simulink model "gm_gm_hdlcoder_commviterbi"  (R2023b)
settings: Solver=FixedStepDiscrete  StartTime=0.0  StopTime=5000  RelTol=1e-3
InitFcn:
  | EbNo=3;
libraries: commcnvcod2 x2, commrandsrc3 x1, commsink2 x1
Description:
  | Viterbi Decoder Using Simulink(R) Blocks
  | This model shows how to use HDL Coder(TM) to check, generate,
  | and verify HDL for a fixed-point Viterbi decoder model built using Simulink(R) blocks.
settings Model: Creator=The MathWorks, Inc.  LastModifiedBy=bryan
settings SolverCC: AlgebraicLoopSolver=TrustRegion  MaxZcPerStep=1
settings DataIOCC: LimitDataPoints=on  SaveFormat=Array  SaveOutput=off  SignalLogging=off  SaveTime=off  ReturnWorkspaceOutputs=off
settings OptimizationCC: BlockReduction=off  ConditionallyExecuteInputs=off  DefaultParameterBehavior=Inlined  ReuseModelBlockBuffer=off  ExpressionDepthLimit=2147483647  InitFltsAndDblsToZero=on  EfficientMapNaN2IntZero=off  LifeSpan=inf
settings DebuggingCC: AlgebraicLoopMsg=error  SignalResolutionControl=TryResolveAllWithWarning  SolverPrmCheckMsg=warning  InheritedTsInSrcMsg=none  MultiTaskDSMMsg=warning  MultiTaskCondExecSysMsg=none  SingleTaskRateTransMsg=error  IntegerOverflowMsg=none  ParameterPrecisionLossMsg=none  UnconnectedInputMsg=warning  UnconnectedOutputMsg=warning  UnconnectedLineMsg=warning  StateNameClashWarn=warning  SymbolicDimsDataTypeCodeGenerationDiagnostic=none  SFUnexpectedBacktrackingDiag=warning  SFNoUnconditionalDefaultTransitionDiag=warning  SFExecutionAtInitializationDiag=none  IntegerSaturationMsg=none  ArithmeticOperatorsInVariantConditions=warning
settings HardwareCC: ProdBitPerPointer=32  ProdBitPerSizeT=32  ProdBitPerPtrDiffT=32  ProdLargestAtomicFloat=None  ProdIntDivRoundTo=Undefined  ProdEndianess=Unspecified  ProdWordSize=32  ProdHWDeviceType=ASIC/FPGA  ProdEqTarget=off
settings ModelReferenceCC: EnableRefExpFcnMdlSchedulingChecks=on  PropagateSignalLabelsOutOfModel=off
settings SFSimCC: SimUseLocalCustomCode=off  CustomCodeUndefinedFunction=UseInterfaceOnly
settings RTWCC: RTWUseLocalCustomCode=off  DLArmComputeVersion=19.05
settings CodeAppCC: StateflowObjectComments=on
settings GRTTargetCC: TargetLangStandard=C89/C90 (ANSI)  CombineOutputUpdateFcns=off  GRTInterface=on
settings ConfigComp: CovMetricSettings=dw  CovSaveCumulativeToWorkspaceVar=on  CovSaveSingleToWorkspaceVar=on  CovExternalEMLEnable=off  CovSFcnEnable=off

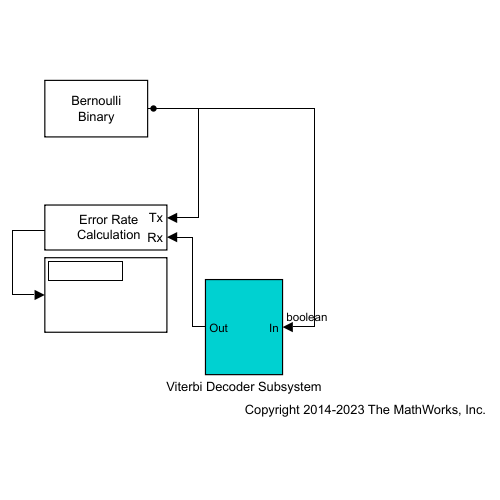
[thumbnail: Simulink's stored preview of the top-level diagram]
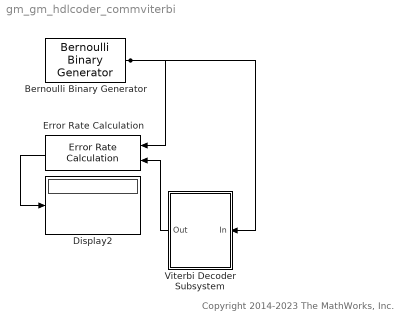
== system gm_gm_hdlcoder_commviterbi ==
  note: Copyright 2014-2023 The MathWorks, Inc.
  Bernoulli Binary Generator : commrandsrc3/Bernoulli Binary Generator  ProbabilityOfZero=0.5  SeedSource=Parameter  Seed=610  SampleTime=1  SamplesPerFrame=1  OutputDataType=boolean  SimulateUsing=Interpreted execution
  Display2 : Display
  Error Rate Calculation : commsink2/Error Rate Calculation  N=32  st_delay=0  cp_mode=Entire frame  subframe=[]  PMode=Port  WsName=BER_Data  RsMode2=off  stop=off  numErr=500  maxBits=1e6
  Viterbi Decoder Subsystem : Subsystem
  wires:
  Bernoulli Binary Generator/1 -> Viterbi Decoder Subsystem/1(In), Error Rate Calculation/1
  Error Rate Calculation/1 -> Display2/1
  Viterbi Decoder Subsystem/1(Out) -> Error Rate Calculation/2

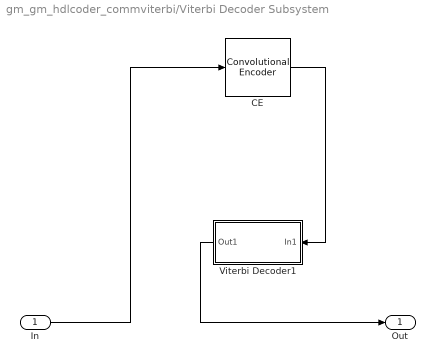
== system gm_gm_hdlcoder_commviterbi/Viterbi Decoder Subsystem ==
  In : Inport  OutDataTypeStr=boolean  PortDimensions=1  SampleTime=1
  CE : commcnvcod2/Convolutional Encoder  trellis=poly2trellis(3,[6 7])  opMode=Continuous  DelayedResetAction=off  hasIniStPort=off  hasFinStPort=off  usePuncVector=off  punctureVector=[1; 1; 0; 1; 0; 1]  reset=Unused parameter value
  Viterbi Decoder1 : Subsystem
  Out : Outport  SampleTime=1  VectorParamsAs1DForOutWhenUnconnected=off
  wires:
  In/1 -> CE/1
  CE/1 -> Viterbi Decoder1/1(In1)
  Viterbi Decoder1/1(Out1) -> Out/1

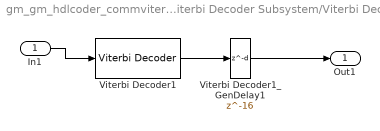
== system gm_gm_hdlcoder_commviterbi/Viterbi Decoder Subsystem/Viterbi Decoder1 ==
  In1 : Inport
  Viterbi Decoder1 : commcnvcod2/Viterbi Decoder  trellis=poly2trellis(3,[6 7])  isPunctured=off  punctureVector=[1; 1; 0; 1; 0; 1]  erasures=off  dectype=Hard decision  nsdecb=3  runSigValErrCheck=off  tbdepth=32  opmode=Continuous  reset=off  delayedResetAction=off  smWordLength=16  outDataType=boolean
  Viterbi Decoder1_GenDelay1 : Delay  DelayLength=16
  Out1 : Outport
  wires:
  In1/1 -> Viterbi Decoder1/1
  Viterbi Decoder1/1 -> Viterbi Decoder1_GenDelay1/1
  Viterbi Decoder1_GenDelay1/1 -> Out1/1
